simulink model "example1"  (R2015b)
settings: Solver=VariableStepAuto  StartTime=0.0  StopTime=tmax  RelTol=1e-3
values from neighbouring files (symbols this model uses):
  A = gamma-alpha    (= 2.5)    [added_current_fitz_relay.m]    (also in example_1.m = [0 1 1; 0 -1 6; 0 0 -1]; getAsymmetricRelayHysteresisForFitzNagumo.m = -0.5; goodwin_prediction.m = [-1 0 0 ; 1 -1 0; 0 1 -1]; new_fitz_relay.m = -1.5)
  B = 1    [added_current_fitz_relay.m]    (also in example_1.m = [1; 6; 6]; getAsymmetricRelayHysteresisForFitzNagumo.m; goodwin_prediction.m = [1; 0 ; 0]; new_fitz_relay.m)
  C = 1    [added_current_fitz_relay.m]    (also in example_1.m = [1 0 0]; getAsymmetricRelayHysteresisForFitzNagumo.m; goodwin_prediction.m = [0 0 1]; new_fitz_relay.m)
  epsilon_1 = out(1)    [added_current_fitz_relay.m]    (also in example_1.m = -1; new_fitz_relay.m = -(epsilon_1 - I_app); relay_fitz_nagumo.m = a(1,1))
  epsilon_2 = out(2)    [added_current_fitz_relay.m]    (also in example_1.m = 1; new_fitz_relay.m = -(epsilon_2 - I_app); relay_fitz_nagumo.m = a(1,3))
  X0 = a1    [added_current_fitz_relay.m]    (also in example_1.m; new_fitz_relay.m; relay_fitz_nagumo.m = a2; test_goodwin.m = -a1)
settings Model: Creator=rajiv  LastModifiedBy=rajiv

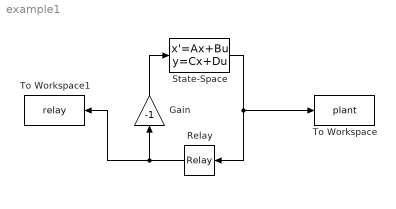
== system example1 ==
  Gain : Gain  Gain=-1
  Relay : Relay  OnSwitchValue=epsilon_2  OffSwitchValue=epsilon_1  OffOutputValue=-1
  State-Space : StateSpace  A=A  B=B  C=C  D=0  X0=X0
  To Workspace : ToWorkspace  VariableName=plant  SaveFormat=Timeseries  SampleTime=-1
  To Workspace1 : ToWorkspace  VariableName=relay  SaveFormat=Timeseries  SampleTime=-1
  wires:
  State-Space/1 -> Relay/1, To Workspace/1
  Relay/1 -> To Workspace1/1, Gain/1
  Gain/1 -> State-Space/1
